simulink model "Automated_features1"  (R2020b)
settings: Solver=VariableStepAuto  StartTime=0.0  StopTime=10.0  RelTol=1e-3
undefined symbols (not defined in the file): sigbuilder_block
libraries: simulink x126
(part 3 of 3)

== stateflow chart Automated_features1/MODULES/ALARM_SYSTEM/ARMED ==
  state data
  state DELAY_1
    entry:
    data1 = 1;
  state DELAY
    entry:
    count=0;
    count = count + 1;
    data1 = 1;
  data -> DELAY_1 [order 2] : [data==1]
  (default) -> data
  data -> DELAY [order 1] : [data==0]
  DELAY -> DELAY : [count~=30]
  data: data input; data1 output; count local

== stateflow chart Automated_features1/MODULES/ALARM_SYSTEM/Main_Alarm/ARMED ==
  state data
  state DELAY_1
    entry:
    data1 = 1;
  state DELAY
    entry:
    count=0;
    count = count + 1;
    data1 = 1;
  data -> DELAY_1 [order 2] : [data==1]
  (default) -> data
  data -> DELAY [order 1] : [data==0]
  DELAY -> DELAY : [count~=30]
  data: data input; data1 output; count local

== stateflow chart Automated_features1/MODULES/ALARM_SYSTEM/Main_Alarm/Pre_Alarm ==
  state RKE1
    entry:
  state DELAY_3
    entry:
    data1 = 1;
  state DELAY_2
    entry:
    counter=0;
    counter = counter +1;
    data1 = 0;
  (default) -> RKE1
  RKE1 -> DELAY_3 [order 2] : [data==1]
  RKE1 -> DELAY_2 [order 1] : [data==0]
  DELAY_2 -> DELAY_2 : [counter~=10]
  data: data input; data1 output; counter local

== stateflow chart Automated_features1/MODULES/ALARM_SYSTEM/Pre_Alarm ==
  state RKE1
    entry:
  state DELAY_3
    entry:
    data1 = 1;
  state DELAY_2
    entry:
    counter=0;
    counter = counter +1;
    data1 = 0;
  (default) -> RKE1
  RKE1 -> DELAY_3 [order 2] : [data==1]
  RKE1 -> DELAY_2 [order 1] : [data==0]
  DELAY_2 -> DELAY_2 : [counter~=10]
  data: data input; data1 output; counter local
